simulink model "PSO_MPPT"  (R2020a)
settings: Solver=VariableStepAuto  StartTime=0.0  StopTime=2.5  MaxStep=1e-4  RelTol=1e-3
libraries: powerlib x16, re_lib x4, powerlib_meascontrol x1
settings Model: Creator=Mahesh Krishna  LastModifiedBy=ADMIN
settings DataIOCC: ReturnWorkspaceOutputs=off
settings OptimizationCC: LifeSpan=inf
settings DebuggingCC: ArithmeticOperatorsInVariantConditions=warning
settings SFSimCC: SimUseLocalCustomCode=off  CustomCodeUndefinedFunction=UseInterfaceOnly
settings RTWCC: RTWUseLocalCustomCode=off
settings CodeAppCC: StateflowObjectComments=on
settings SimscapeCC: SimscapeNormalizeSystem=off

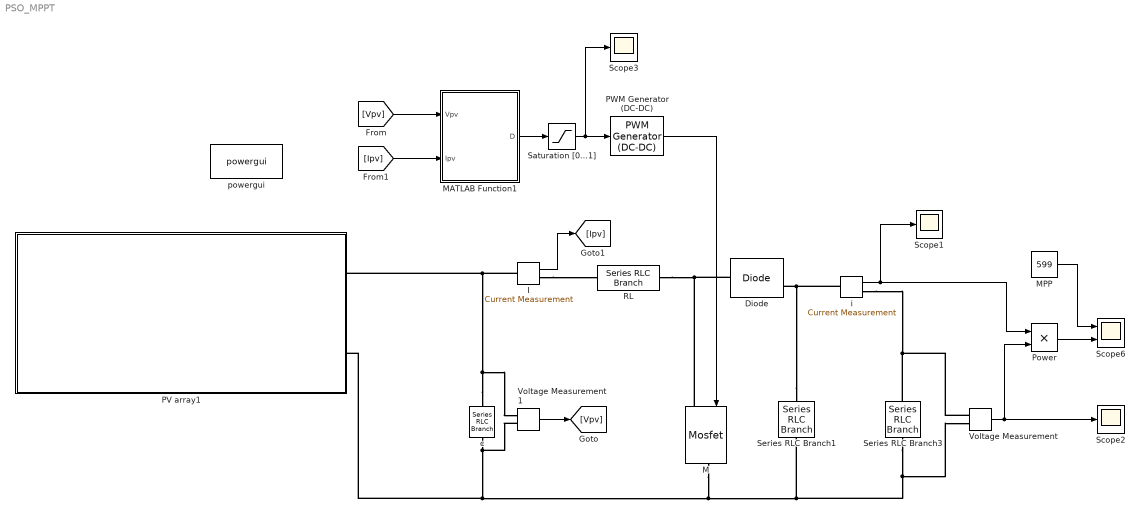
== system PSO_MPPT ==
  Diode : powerlib/Power Electronics/Diode  Ron=1e-3  Lon=0  Vf=0  IC=0  UseSnubber=0  Rs=inf  Cs=inf  Measurements=on
  I : powerlib/Measurements/Current Measurement  PhasorSimulation=off  OutputType=Magnitude  PSBequivalent=0
  M : powerlib/Power Electronics/Mosfet  Ron=1e-3  Lon=0  Rd=1e-3  Vfd=0  IC=0  Rs=inf  Cs=inf  Measurements=off
  MATLAB Function1 : MATLAB Function  TreatAsAtomicUnit=on
  MPP : Constant  Value=599
  PV array1 : Subsystem
  PWM Generator (DC-DC) : powerlib_meascontrol/Pulse & Signal Generators/PWM Generator (DC-DC)  Fsw=50e3  Ts=0
  Power : Product
  RL : powerlib/Elements/Series RLC Branch  LConnTagsString=__new0  RConnTagsString=__new0  BranchType=L  Resistance=1e-3  Inductance=0.0012  SetiL0=off  InitialCurrent=0  Capacitance=1e-6  Setx0=off  InitialVoltage=0  Measurements=None
  Saturation [0...1] : Saturate  UpperLimit=1  LowerLimit=0
  Scope1 : Scope
  Scope2 : Scope
  Scope3 : Scope
  Scope6 : Scope  NumInputPorts=2
  Series RLC Branch1 : powerlib/Elements/Series RLC Branch  LConnTagsString=__new0  RConnTagsString=__new0  BranchType=C  Resistance=1e-4  Inductance=200e-6  SetiL0=off  InitialCurrent=0  Capacitance=0.4676e-3  Setx0=off  InitialVoltage=40  Measurements=None
  Series RLC Branch3 : powerlib/Elements/Series RLC Branch  LConnTagsString=__new0  RConnTagsString=__new0  BranchType=R  Resistance=58  Inductance=200e-6  SetiL0=off  InitialCurrent=0  Capacitance=1000e-6  Setx0=off  InitialVoltage=40  Measurements=None
  Voltage Measurement : powerlib/Measurements/Voltage Measurement  PhasorSimulation=off  OutputType=Magnitude  PSBequivalent=0
  Voltage Measurement1 : powerlib/Measurements/Voltage Measurement  PhasorSimulation=off  OutputType=Magnitude  PSBequivalent=0
  c : powerlib/Elements/Series RLC Branch  LConnTagsString=__new0  RConnTagsString=__new0  BranchType=C  Resistance=1e-3  Inductance=250e-6  SetiL0=off  InitialCurrent=0  Capacitance=10e-6  Setx0=off  InitialVoltage=0  Measurements=None
  i : powerlib/Measurements/Current Measurement  PhasorSimulation=off  OutputType=Magnitude  PSBequivalent=0
  powergui : powerlib/powergui  Priority=1  SimulationMode=Continuous  SampleTime=50e-6  frequency=60  Iterations=50  frequencyindice=0  Pbase=100e6  ErrMax=1e-4  UnitsV=kV  UnitsW=MW  buscounter=0  FunctionMessages=off  echomessages=off  EnableUseOfTLC=off  CurrentSourceSwitches=off  DisableSnubberDevices=off  DisableRonSwitches=off  DisableVfSwitches=off  DisplayEquations=off  AutomaticDiscreteSolvers=off  SolverType=Tustin/Backward Euler (TBE)  Interpol=off  ExternalGateDelay=off  methode=off  Ts=100  x0status=blocks  SPID=on  SwTol=0  HookPort=off  NonlinearTolerance=1e-4  nMaxIteration=100  ContinueOnMaxIteration=off  RestoreLinks=warning  ResistiveCurrentMeasurement=off  Frange=[0:2:500]  Ylog=off  Xlog=on  ShowGrid=off  save=off  variable=ZData  structure=0  ZoomFFT=off  StartTime=0.0  cycles=1  DisplayStyle=1  fundamental=60  FreqAxis=off  MaxFrequency=1000  frequencyindicesteady=1  RmsSteady=1  display=off
  wires:
  I/1 -> [Ipv]
  [Ipv] -> MATLAB Function1/2(Ipv)
  Voltage Measurement/1 -> Scope2/1, Power/2
  MATLAB Function1/1(D) -> Saturation [0...1]/1
  PWM Generator (DC-DC)/1 -> M/1
  i/1 -> Scope1/1, Power/1
  Saturation [0...1]/1 -> Scope3/1, PWM Generator (DC-DC)/1
  Voltage Measurement1/1 -> [Vpv]
  [Vpv] -> MATLAB Function1/1(Vpv)
  MPP/1 -> Scope6/1
  Power/1 -> Scope6/2
  connections:
  i/RConn1 -- Series RLC Branch3/LConn1 -- Voltage Measurement/LConn1
  Series RLC Branch3/RConn1 -- M/RConn1 -- Voltage Measurement1/LConn2 -- c/RConn1 -- PV array1/RConn2 -- Series RLC Branch1/RConn1 -- Voltage Measurement/LConn2
  Series RLC Branch1/LConn1 -- i/LConn1 -- Diode/RConn1
  c/LConn1 -- I/LConn1 -- PV array1/RConn1 -- Voltage Measurement1/LConn1
  M/LConn1 -- RL/RConn1 -- Diode/LConn1
  I/RConn1 -- RL/LConn1

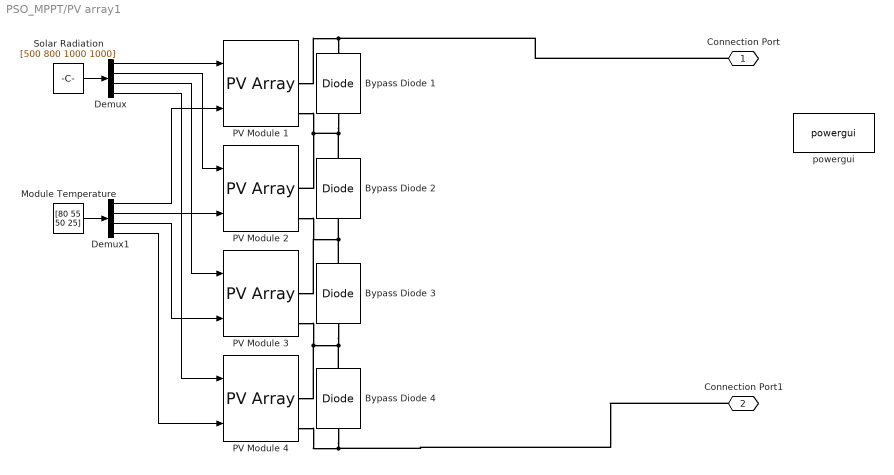
== system PSO_MPPT/PV array1 ==
  Bypass Diode {1..4} (4 alike) : powerlib/Power Electronics/Diode  Ron=0.001  Lon=0  Vf=0.8  IC=0  UseSnubber=off  Rs=500  Cs=250e-9  Measurements=off
  Demux : Demux
  Demux1 : Demux
  Module Temperature : Constant  Value=[80 55 50 25]
  PV Module {1..4} (4 alike) : re_lib/Solar/PV Array  Npar=1  Nser=1  PlotType=array @ 1000 W/m2 & specified temperatures  S_vec="[ 1000  500  100 ]"  Temp_C_vec="[ 45 25  ]"  ModuleName=Tata Power Solar Systems TP250MBZ  PlotWhenSelected=off  Pm=249  Ncell=60  Voc=36.8  Isc=8.83  Vm=30  Im=8.3  beta_Voc_pc=-0.33  alpha_Isc_pc=0.063805  beta_Voc=-0.12144  alpha_Isc=0.005634  IL=8.8382  I0=1.0132e-10  nI=0.94812  Rsh=314.7646  Rs=0.2914  RobustModel=off  RobustCellTemperature=25  BAL=off  Tc=1e-6  Tfilter=5e-5
  Solar Radiation : Constant  Value=[500 800 1000 1000]
  powergui : powerlib/powergui  Priority=1  SimulationMode=Continuous  SampleTime=50e-6  frequency=60  Iterations=50  frequencyindice=0  Pbase=100e6  ErrMax=1e-4  UnitsV=kV  UnitsW=MW  buscounter=0  FunctionMessages=off  echomessages=off  EnableUseOfTLC=off  CurrentSourceSwitches=off  DisableSnubberDevices=off  DisableRonSwitches=off  DisableVfSwitches=off  DisplayEquations=off  AutomaticDiscreteSolvers=off  SolverType=Tustin/Backward Euler (TBE)  Interpol=off  ExternalGateDelay=off  methode=off  Ts=100  x0status=blocks  SPID=on  SwTol=0  HookPort=off  NonlinearTolerance=1e-4  nMaxIteration=100  ContinueOnMaxIteration=off  RestoreLinks=warning  ResistiveCurrentMeasurement=off  Frange=[0:2:500]  Ylog=off  Xlog=on  ShowGrid=off  save=off  variable=ZData  structure=0  ZoomFFT=off  StartTime=0.0  cycles=1  DisplayStyle=1  fundamental=60  FreqAxis=off  MaxFrequency=1000  frequencyindicesteady=1  RmsSteady=1  display=off
  Connection Port : PMIOPort  Side=Right
  Connection Port1 : PMIOPort  Port=2  Side=Right
  wires:
  Solar Radiation/1 -> Demux/1
  Demux1/4 -> PV Module 4/2
  Demux/2 -> PV Module 2/1
  Module Temperature/1 -> Demux1/1
  Demux/3 -> PV Module 3/1
  Demux1/2 -> PV Module 2/2
  Demux/1 -> PV Module 1/1
  Demux1/1 -> PV Module 1/2
  Demux1/3 -> PV Module 3/2
  Demux/4 -> PV Module 4/1
  connections:
  Bypass Diode 3/RConn1 -- Bypass Diode 2/LConn1 -- PV Module 2/RConn2 -- PV Module 3/RConn1
  PV Module 3/RConn2 -- Bypass Diode 4/RConn1 -- Bypass Diode 3/LConn1 -- PV Module 4/RConn1
  Bypass Diode 2/RConn1 -- Bypass Diode 1/LConn1 -- PV Module 2/RConn1 -- PV Module 1/RConn2
  PV Module 1/RConn1 -- Connection Port/RConn1 -- Bypass Diode 1/RConn1
  Bypass Diode 4/LConn1 -- Connection Port1/RConn1 -- PV Module 4/RConn2

== matlab function PSO_MPPT/MATLAB Function1 ==
  settings: updateMethod=DISCRETE  sampleTime=1e-4
  data: Vpv input; D output; Ipv input
function D = PSO(Vpv,Ipv)
%Initialization
%= u = index of current particle, dcurrent = current duty cycle, 
%pbest = personal best dc value, p= power of pos, v=velocity
% dc = duty cycle of pos, counter to limit duty cycles update(interation)
persistent u dcurrent pbest p dc v counter gbest;

if(isempty(counter))
    counter=0;
end
if(isempty(dcurrent))
    dcurrent=0.5;
end
if(isempty(gbest))
    gbest=0.5;
end
if(isempty(p))
    p=zeros(4,1);
end

if(isempty(v))
    v=zeros(4,1);
end

if(isempty(pbest))
    pbest=zeros(4,1);
end
if(isempty(u))
    u=0;
end
if(isempty(dc))
    dc=zeros(4,1);
    dc(1)=0;
    dc(2)=0.3;
    dc(3)=0.5;
    dc(4)=0.9;
end
if(counter>=1 && counter<300)
    D=dcurrent;
    counter=counter+1;
    return;
end
counter=0;
%goes through each particle, if Vpv*Ipv is greater than current particle's
%p, current bet position is updated
if(u>=1 && u<=4)
    if((Vpv*Ipv)>p(u))
        p(u)=Vpv*Ipv;
        pbest(u)=dcurrent;
    end
end
u=u+1;
if(u==6)
    u=1;
end
if(u==1)
    D=dc(u);
    dcurrent=D;
    counter=1;
    return;
elseif(u==2)
    D=dc(u);
    dcurrent=D;
    counter=1;
    return;
elseif(u==3)
    D=dc(u);
    dcurrent=D;
    counter=1;
    return;
elseif(u==4)
    D=dc(u);
    dcurrent=D;
    counter=1;
    return;
elseif(u==5 ) %at u=5, retrieve the best duty cycle, set best position to global best 
    [m,i]=max(p);
    gbest=pbest(i);
    D=gbest; %assign gbest to D
    dcurrent=D; %assign D to current dc
    counter=1;
    
    %update velocity and duty cycle
    v(1)=updatevelocity(v(1),pbest(1),dc(1),gbest)
    v(2)=updatevelocity(v(2),pbest(2),dc(2),gbest)
    v(3)=updatevelocity(v(3),pbest(3),dc(3),gbest)
    v(4)=updatevelocity(v(4),pbest(4),dc(4),gbest)
    %update duty cycle
    dc(1)=updateduty(dc(1),v(1))
    dc(2)=updateduty(dc(2),v(2))
    dc(3)=updateduty(dc(3),v(3))
    dc(4)=updateduty(dc(4),v(4))
    
    return;
    
else
    u
    y='hhahah'
    D=0.1
    
end


end
function vfinal=updatevelocity(velocity,pobest,d,gwbest)
% PSO Parameters
w=0.4; 
%w=(1.1-(pobest/gwbest));            % Inertia Weight
             % Inertia Weight Damping Ratio
c1= 1.2;         % Personal Learning Coefficient
c2=1.2;         % Global Learning Coefficient
k1 =rand(1); 
k2 =rand(1);
vfinal = (w*velocity)+(c1*k1*(pobest-d))+(c2*k2*(gwbest-d));
end

function dfinal=updateduty(d,velocity)
dup=d+velocity;
if(dup>1)
    dfinal=1;
elseif(dup<0)
    dfinal=0;
else
    dfinal=dup;
end
end
